simulink model "am_2"  (Simulink 4.00)
settings: Solver=ode45  StartTime=0  StopTime=5  RelTol=1e-3
undefined symbols (not defined in the file or in its folder): B, fmax, fn, Fs, get, k
libraries: dspindex x4, dsparch3 x3, dspsnks3 x3, dspmtrx3 x3, dspsigattribs x2, dspspect3 x2, simulink3 x2, dspbuff3 x2, dspmathops x2, commsource2 x1
Description:
  | Model lacza cyfrowego z modulacja ASK/FSK/PSK
settings Model: Creator=Tomas  LimitDataPoints=off  MaxDataPoints=10000  RTWOptions="-aEnforceIntegerDowncast=1 -aExtMode=0 -aFoldNonRolledExpr=1 -aForceParamTrailComments=0 -aGenerateComments=1 -aIgnoreCustomStorageClasses=1 -aIncHierarchyInIds=0 -aInlineInvariantSignals=0 -aLocalBlockOutputs=1 -aLogVarNameModifier=\"rt_\" -aRTWVerbose=1 -aRollThreshold=5 -aShowEliminatedStatements=1"  RTWInlineParameters=on  BlockReductionOpt=off

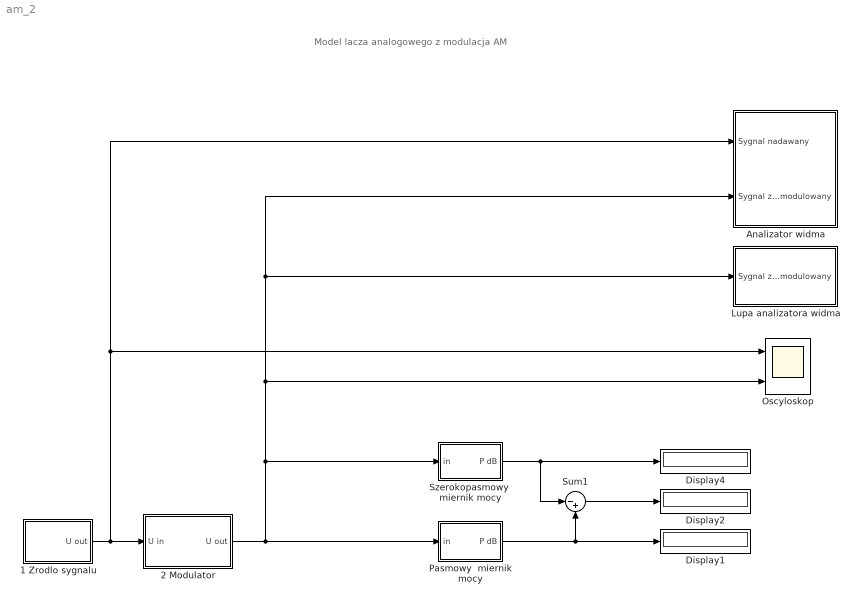
== system am_2 ==
  note: Model lacza analogowego z modulacja AM
  1 Zrodlo sygnalu : Subsystem  mask(Źródło sygnału){on=on, sq=off, bity=100}
      mask prompts: on "Włączenie źródła sygnału"; sq "Przebieg losowy"; bity "częstotliwość/pasmo"
      mask help:
      | Generuje sygnał testowy.
      | Moc wyjściowa 0 dB.
      mask init:
      | if (sq == 0) sq = 1;
      | else sq = 0;
      | end;
      | if (on == 0)
      | set_param(gcb,'MaskEnables',{,'on','off','off'}); fgen=100; G=1;
      | else
      |   set_param(gcb,'MaskEnables',{,'on','on','on'});
      |   if (bity == 1) fgen = 100; G=1/0.1791;
      |   elseif (bity == 2) fgen = 200; G=1/0.2467;
      |   else fgen = 300; G=1/0.3022;
      |   end;
      | end;
      settings: RTWFcnNameOpts=Auto  RTWFileNameOpts=Auto
      mask Help: No help
      mask StyleString: checkbox,checkbox,popup(100|200|300)
      mask Display: disp('Sygnal\nnadawany')
  2 Modulator : Subsystem  mask(Modulator AM){on=on, p=0.7}
      mask prompts: on "Włączenie modulatora"; p "Głębokość modulacji (0..1):"
      mask help:
      | Dokonuje operacji modulacji AM sygnałem podanym na wejście.
      | Częstotliość nośnej: 1000 Hz.
      mask init:
      | fnos=1000;
      | if (on==0) k=1; set_param(gcb,'MaskEnables',{,'on','off'});
      | else set_param(gcb,'MaskEnables',{,'on','on'});
      |   if (p == 1) k = 0.1;
      |   elseif (p == 2) k = 0.2;
      |   elseif (p == 3) k = 0.3;
      |   elseif (p == 4) k = 0.4;
      |   elseif (p == 5) k = 0.5;
      |   elseif (p == 6) k = 0.6;
      |   elseif (p == 7) k = 0.7;
      |   elseif (p == 8) k = 0.8;
      |   elseif (p == 9) k = 0.9;
      |   elseif (p == 10) k = 1.0;
      |   else k = 1.5;
      |   end;
      | end;
      | on=on+1;
      settings: RTWFcnNameOpts=Auto  RTWFileNameOpts=Auto
      mask Help: No help
      mask StyleString: checkbox,popup(0.1|0.2|0.3|0.4|0.5|0.6|0.7|0.8|0.9|1.0|1.5)
      mask Display: disp('Modulator\nAM')
  "Analizator widma " : Subsystem
      settings: RTWFcnNameOpts=Auto  RTWFileNameOpts=Auto
  Display1 : Display
      settings: Format=short
  Display2 : Display
      settings: Format=short
  Display4 : Display
      settings: Format=short
  Lupa analizatora widma : Subsystem  mask(Analizator){f=....fo+1000Hz}
      mask prompts: f "zakres częstotliwości:   fo.."
      mask help: Analizator widma o regulowanym zakresie względem fo=1000Hz
      mask init:
      | if (f==1) fmax=64; elseif (f==2) fmax=128; elseif (f==3) fmax=256; elseif (f==4) fmax=512; else fmax=1024; end;
      settings: RTWFcnNameOpts=Auto  RTWFileNameOpts=Auto
      mask StyleString: popup(....fo+50Hz|....fo+100Hz|....fo+250Hz|....fo+500Hz|....fo+1000Hz)
      mask Display: disp('Lupa')
  Oscyloskop : Scope  NumInputPorts=2
      settings: TimeRange=1  YMin=0~-7.5  YMax=1~7.5  SaveToWorkspace=off  DataFormat=Array  MaxDataPoints=10000
  Pasmowy  miernik mocy : Subsystem  mask(Pasmowy miernik mocy (RMS)){B=200, ca=on, av=on}
      mask prompts: B "pasmo [Hz]"; ca "odfiltruj nośną (1000Hz)"; av "uśrednianie (max. 5 próbek)"
      mask help:
      | Pasmowy miernik mocy (RMS).
      | Częstotliwość środkowa pasma 1000 Hz.
      mask init:
      | fn=1000;
      | BufferSize=4096*8;
      | MaxIndex=BufferSize/2+1;
      | if (B/2<=fn) LowIndex=round(fn-B/2)+1; else LowIndex=1; end;
      | if( B/2+fn<=BufferSize/2) HighIndex=round(fn+B/2)+1; else HighIndex=MaxIndex; end;
      | if (ca==1) ca1_mi_de=round(fn)-3; ca1_pl_de=round(fn)+3;
      | else ca1_mi_de=LowIndex+1; ca1_pl_de=ca1_mi_de+1; end;
      settings: RTWFcnNameOpts=Auto  RTWFileNameOpts=Auto
  Sum1 : Sum  Inputs=|-+  SaturateOnIntegerOverflow=on
  Szerokopasmowy  miernik mocy : Subsystem  mask(Szerokopasmowy miernik mocy (RMS)){ca=on, av=on}
      mask prompts: ca "odfiltruj nośną (1000Hz)"; av "uśrednianie (max 5 próbek)"
      mask help: Szerokopasmowy miernik mocy (RMS).
      mask init:
      | fn=1000;
      | BufferSize=4096*8;
      | MaxIndex=BufferSize/2+1;
      | LowIndex=1;
      | HighIndex=MaxIndex;
      | if (ca==1) ca1_mi_de=round(fn)-3; ca1_pl_de=round(fn)+3;
      | else ca1_mi_de=LowIndex+1; ca1_pl_de=ca1_mi_de+1; end;
      settings: RTWFcnNameOpts=Auto  RTWFileNameOpts=Auto
  wires:
  2 Modulator/1(U out) -> "Analizator widma "/2(Sygnal zmodulowany), Lupa analizatora widma/1(Sygnal zmodulowany), Oscyloskop/2, Szerokopasmowy  miernik mocy/1(in), Pasmowy  miernik mocy/1(in)
  1 Zrodlo sygnalu/1(U out) -> "Analizator widma "/1(Sygnal nadawany), Oscyloskop/1, 2 Modulator/1(U in)
  Sum1/1 -> Display2/1
  Pasmowy  miernik mocy/1(P dB) -> Sum1/2, Display1/1
  Szerokopasmowy  miernik mocy/1(P dB) -> Display4/1, Sum1/1

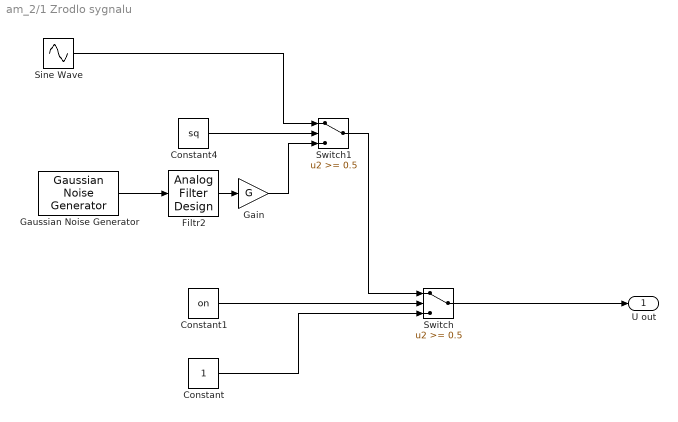
== system am_2/1 Zrodlo sygnalu ==
  Constant : Constant  Value=1
  Constant1 : Constant  Value=on
  Constant4 : Constant  Value=sq
  Filtr2 : dsparch3/Analog Filter Design  method=Chebyshev II  filttype=Lowpass  N=16  Wlo=2*pi*fgen  Whi=2*pi*(fn+B/2)  Rp=2  Rs=60
  Gain : Gain  Gain=G  Multiplication=Element-wise(K.*u)  SaturateOnIntegerOverflow=on
  Gaussian Noise Generator : commsource2/Gaussian Noise Generator  m=0  d=1  s=12345  Ts=1/(6000)  frameBased=off  sampPerFrame=1  orient=off
  Sine Wave : Sin  SineType=Time-based  Amplitude=sqrt(2)  Bias=0  Frequency=2*pi*fgen  Phase=0  Samples=10  SampleTime=0  Offset=0
  Switch : Switch  Threshold=0.5
  Switch1 : Switch  Threshold=0.5
  U out : Outport  Port=1
  wires:
  Switch/1 -> U out/1
  Constant1/1 -> Switch/2
  Switch1/1 -> Switch/1
  Constant4/1 -> Switch1/2
  Sine Wave/1 -> Switch1/1
  Constant/1 -> Switch/3
  Gaussian Noise Generator/1 -> Filtr2/1
  Filtr2/1 -> Gain/1
  Gain/1 -> Switch1/3

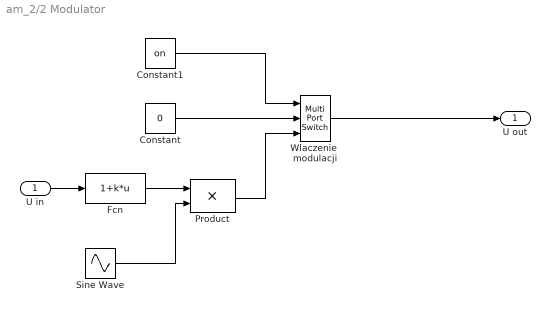
== system am_2/2 Modulator ==
  U in : Inport  Port=1  LatchInput=off
  Constant : Constant  Value=0
  Constant1 : Constant  Value=on
  Fcn : Fcn  Expr=1+k*u
  Product : Product  Inputs=2  Multiplication=Element-wise(.*)  SaturateOnIntegerOverflow=on
  Sine Wave : Sin  SineType=Time-based  Amplitude=1  Bias=0  Frequency=2*pi*1000  Phase=0  Samples=10  SampleTime=0  Offset=0
  Wlaczenie  modulacji : MultiPortSwitch  Inputs=2
  U out : Outport  Port=1
  wires:
  Wlaczenie  modulacji/1 -> U out/1
  Constant1/1 -> Wlaczenie  modulacji/1
  Constant/1 -> Wlaczenie  modulacji/2
  Product/1 -> Wlaczenie  modulacji/3
  U in/1 -> Fcn/1
  Fcn/1 -> Product/1
  Sine Wave/1 -> Product/2

== system am_2/Analizator widma  ==
  Sygnal nadawany : Inport  Port=1  LatchInput=off
  Sygnal zmodulowany : Inport  Port=2  LatchInput=off
  "Sygnal nadawany " : dspsnks3/Spectrum Scope  ScopeProperties=on  Domain=Frequency  HorizSpan=1  UseBuffer=on  BufferSize=4096  Overlap=0  inpFftLenInherit=off  FFTlength=128  numAvg=1  DisplayProperties=off  AxisGrid=on  Memory=on  FrameNumber=off  AxisLegend=off  AxisZoom=off  OpenScopeAtSimStart=on  OpenScopeImmediately=off  FigPos=get(0,'defaultfigureposition')  AxisProperties=off  XUnits=Hertz  XRange=[-Fs/2...Fs/2]  InheritXIncr=on  XIncr=1.0  XLabel=Samples  YUnits=dB  YLabel=Magnitude  LineProperties=off  LineMarkers=None
      settings: YMin=-10  YMax=23.8040697044832
  "Sygnal zmodulowany " : dspsnks3/Spectrum Scope  ScopeProperties=on  Domain=Frequency  HorizSpan=1  UseBuffer=on  BufferSize=4096  Overlap=0  inpFftLenInherit=off  FFTlength=128  numAvg=1  DisplayProperties=off  AxisGrid=on  Memory=on  FrameNumber=off  AxisLegend=off  AxisZoom=off  OpenScopeAtSimStart=on  OpenScopeImmediately=off  FigPos=get(0,'defaultfigureposition')  AxisProperties=off  XUnits=Hertz  XRange=[-Fs/2...Fs/2]  InheritXIncr=on  XIncr=1.0  XLabel=Samples  YUnits=dB  YLabel=Magnitude  LineProperties=off  LineMarkers=None
      settings: YMin=-52.7531800625172  YMax=26.1007017107538
  Unit Delay3 : UnitDelay  X0=0  SampleTime=1/4096
      settings: RTWStateStorageClass=Auto
  Unit Delay4 : UnitDelay  X0=0  SampleTime=1/4096
      settings: RTWStateStorageClass=Auto
  wires:
  Unit Delay4/1 -> "Sygnal nadawany "/1
  Sygnal nadawany/1 -> Unit Delay4/1
  Unit Delay3/1 -> "Sygnal zmodulowany "/1
  Sygnal zmodulowany/1 -> Unit Delay3/1

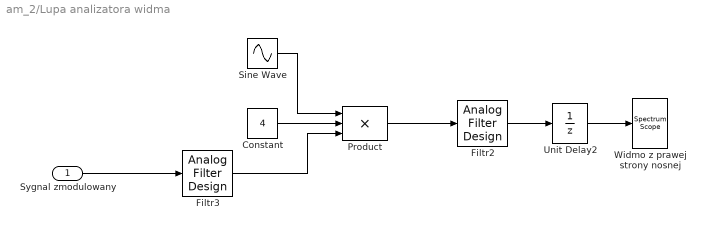
== system am_2/Lupa analizatora widma ==
  Sygnal zmodulowany : Inport  Port=1  LatchInput=off
  Constant : Constant  Value=4
  Filtr2 : dsparch3/Analog Filter Design  method=Elliptic  filttype=Lowpass  N=12  Wlo=2*pi*fmax  Whi=2*pi*(fn+B/2)  Rp=0.2  Rs=80
  Filtr3 : dsparch3/Analog Filter Design  method=Elliptic  filttype=Lowpass  N=26  Wlo=2*pi*1000  Whi=2*pi*(fn+B/2)  Rp=0.2  Rs=80
  Product : Product  Inputs=3  Multiplication=Element-wise(.*)  SaturateOnIntegerOverflow=off
  Sine Wave : Sin  SineType=Time-based  Amplitude=1  Bias=0  Frequency=2*pi*1000  Phase=2*pi-0.03*pi  Samples=10  SampleTime=0  Offset=0
  Unit Delay2 : UnitDelay  X0=0  SampleTime=1/(2*fmax)
      settings: RTWStateStorageClass=Auto
  Widmo z prawej strony nosnej : dspsnks3/Spectrum Scope  ScopeProperties=on  Domain=Frequency  HorizSpan=1  UseBuffer=on  BufferSize=2*fmax  Overlap=0  inpFftLenInherit=off  FFTlength=128  numAvg=1  DisplayProperties=off  AxisGrid=on  Memory=on  FrameNumber=off  AxisLegend=off  AxisZoom=off  OpenScopeAtSimStart=on  OpenScopeImmediately=off  FigPos=get(0,'defaultfigureposition')  AxisProperties=off  XUnits=Hertz  XRange=[0...Fs/2]  InheritXIncr=on  XIncr=1.0  XLabel=Samples  YUnits=dB  YLabel=Magnitude  LineProperties=off  LineMarkers=None
      settings: YMin=-30  YMax=20
  wires:
  Sine Wave/1 -> Product/1
  Product/1 -> Filtr2/1
  Sygnal zmodulowany/1 -> Filtr3/1
  Constant/1 -> Product/2
  Unit Delay2/1 -> Widmo z prawej strony nosnej/1
  Filtr3/1 -> Product/3
  Filtr2/1 -> Unit Delay2/1

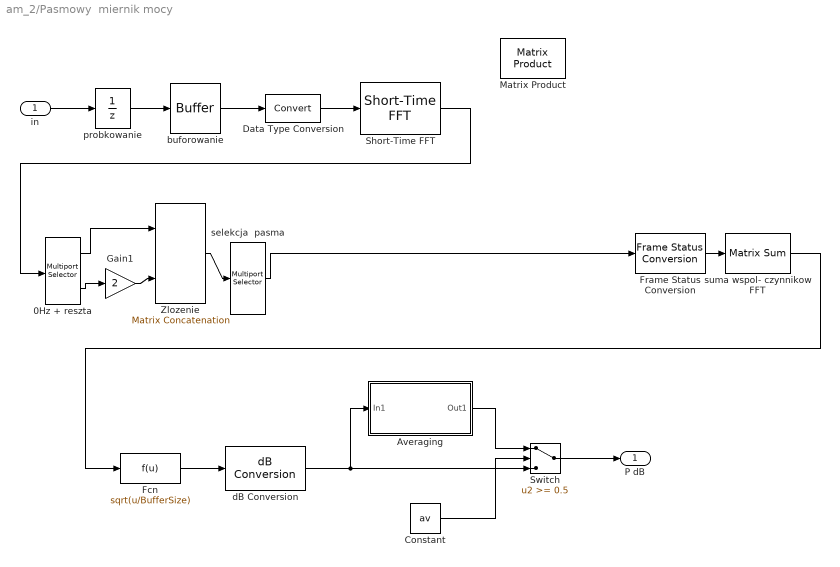
== system am_2/Pasmowy  miernik mocy ==
  in : Inport  Port=1  LatchInput=off
  0Hz + reszta : dspindex/Multiport Selector  rowsOrCols=Rows  idxCellArray={[1],[2:MaxIndex]}  idxErrMode=Generate Error
  Averaging : Subsystem
      settings: RTWFcnNameOpts=Auto  RTWFileNameOpts=Auto
  Constant : Constant  Value=av
  Data Type Conversion : DataTypeConversion  DataType=double  SaturateOnIntegerOverflow=on
  Fcn : Fcn  Expr=sqrt(u/BufferSize)
  Frame Status Conversion : dspsigattribs/Frame Status Conversion  growRefPort=off  outframe=Sample-based
  Gain1 : Gain  Gain=2  Multiplication=Element-wise(K.*u)  SaturateOnIntegerOverflow=on
  Matrix Product : dspmtrx3/Matrix Product  Dim=Columns
  Short-Time FFT : dspspect3/Short-Time FFT  wintype=Hann  Rs=50  beta=5  winsamp=Symmetric  inheritFFT=on  fftsize=FFTlength  navg=1
  Switch : Switch  Threshold=0.5
  Zlozenie : simulink3/Signals & Systems/Matrix Concatenation  numInports=2  catMethod=Vertical
  buforowanie : dspbuff3/Buffer  N=BufferSize  V=0  ic=0
  dB Conversion : dspmathops/dB Conversion  dBtype=dB  intype=Amplitude  R=1  fuzz=on
  probkowanie : UnitDelay  X0=0  SampleTime=1/BufferSize
      settings: RTWStateStorageClass=Auto
  selekcja  pasma : dspindex/Multiport Selector  rowsOrCols=Rows  idxCellArray={[LowIndex:ca1_mi_de ca1_pl_de:HighIndex]}  idxErrMode=Generate Error
  suma wspol- czynnikow FFT : dspmtrx3/Matrix Sum  Dim=Columns
  P dB : Outport  Port=1
  wires:
  Data Type Conversion/1 -> Short-Time FFT/1
  buforowanie/1 -> Data Type Conversion/1
  Frame Status Conversion/1 -> suma wspol- czynnikow FFT/1
  probkowanie/1 -> buforowanie/1
  0Hz + reszta/2 -> Gain1/1
  0Hz + reszta/1 -> Zlozenie/1
  Gain1/1 -> Zlozenie/2
  Zlozenie/1 -> selekcja  pasma/1
  selekcja  pasma/1 -> Frame Status Conversion/1
  Short-Time FFT/1 -> 0Hz + reszta/1
  suma wspol- czynnikow FFT/1 -> Fcn/1
  in/1 -> probkowanie/1
  Fcn/1 -> dB Conversion/1
  Averaging/1(Out1) -> Switch/1
  Switch/1 -> P dB/1
  Constant/1 -> Switch/2
  dB Conversion/1 -> Averaging/1(In1), Switch/3

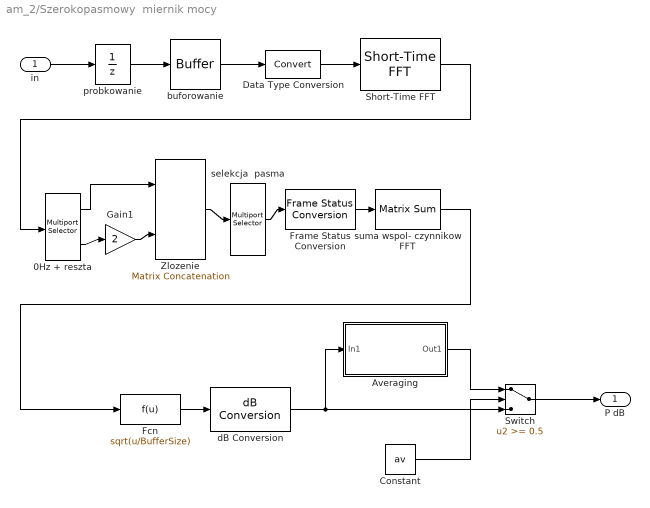
== system am_2/Szerokopasmowy  miernik mocy ==
  in : Inport  Port=1  LatchInput=off
  0Hz + reszta : dspindex/Multiport Selector  rowsOrCols=Rows  idxCellArray={[1],[2:MaxIndex]}  idxErrMode=Generate Error
  Averaging : Subsystem
      settings: RTWFcnNameOpts=Auto  RTWFileNameOpts=Auto
  Constant : Constant  Value=av
  Data Type Conversion : DataTypeConversion  DataType=double  SaturateOnIntegerOverflow=on
  Fcn : Fcn  Expr=sqrt(u/BufferSize)
  Frame Status Conversion : dspsigattribs/Frame Status Conversion  growRefPort=off  outframe=Sample-based
  Gain1 : Gain  Gain=2  Multiplication=Element-wise(K.*u)  SaturateOnIntegerOverflow=on
  Short-Time FFT : dspspect3/Short-Time FFT  wintype=Hann  Rs=50  beta=5  winsamp=Symmetric  inheritFFT=on  fftsize=FFTlength  navg=1
  Switch : Switch  Threshold=0.5
  Zlozenie : simulink3/Signals & Systems/Matrix Concatenation  numInports=2  catMethod=Vertical
  buforowanie : dspbuff3/Buffer  N=BufferSize  V=0  ic=0
  dB Conversion : dspmathops/dB Conversion  dBtype=dB  intype=Amplitude  R=1  fuzz=on
  probkowanie : UnitDelay  X0=0  SampleTime=1/BufferSize
      settings: RTWStateStorageClass=Auto
  selekcja  pasma : dspindex/Multiport Selector  rowsOrCols=Rows  idxCellArray={[LowIndex:ca1_mi_de ca1_pl_de:HighIndex]}  idxErrMode=Generate Error
  suma wspol- czynnikow FFT : dspmtrx3/Matrix Sum  Dim=Columns
  P dB : Outport  Port=1
  wires:
  Data Type Conversion/1 -> Short-Time FFT/1
  buforowanie/1 -> Data Type Conversion/1
  Frame Status Conversion/1 -> suma wspol- czynnikow FFT/1
  probkowanie/1 -> buforowanie/1
  0Hz + reszta/2 -> Gain1/1
  0Hz + reszta/1 -> Zlozenie/1
  Gain1/1 -> Zlozenie/2
  Zlozenie/1 -> selekcja  pasma/1
  selekcja  pasma/1 -> Frame Status Conversion/1
  Short-Time FFT/1 -> 0Hz + reszta/1
  suma wspol- czynnikow FFT/1 -> Fcn/1
  in/1 -> probkowanie/1
  Fcn/1 -> dB Conversion/1
  Averaging/1(Out1) -> Switch/1
  Switch/1 -> P dB/1
  Constant/1 -> Switch/2
  dB Conversion/1 -> Switch/3, Averaging/1(In1)

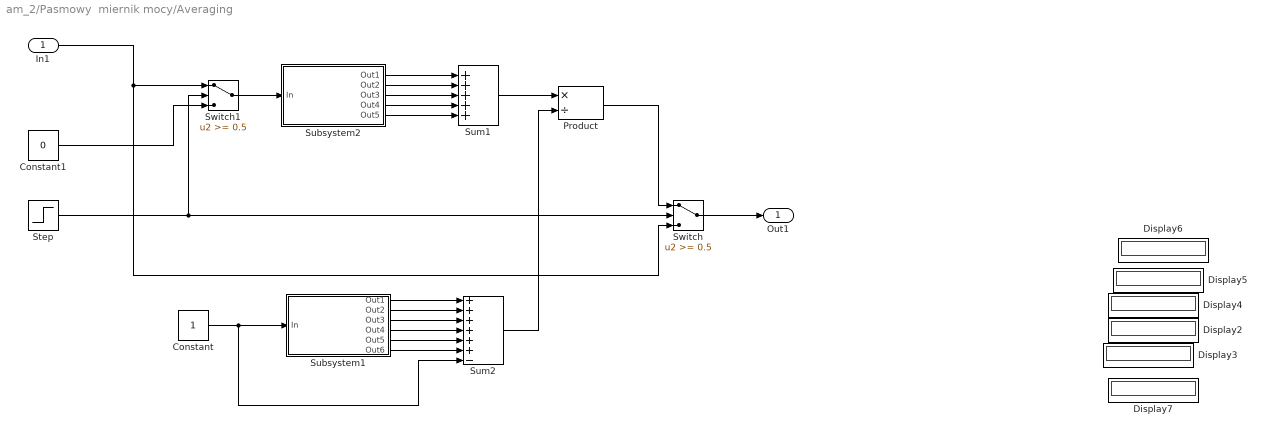
== system am_2/Pasmowy  miernik mocy/Averaging ==
  In1 : Inport  Port=1  LatchInput=off
  Constant : Constant  Value=1
  Constant1 : Constant  Value=0
  Display{2..7} (6 alike) : Display
      settings: Format=short
  Product : Product  Inputs=*/  Multiplication=Element-wise(.*)  SaturateOnIntegerOverflow=on
  Step : Step  Time=1  Before=0  After=1  SampleTime=0
  Subsystem1 : Subsystem  mask(6 Sample Analog Shift Register){tp=1}
      mask prompts: tp "Sample time"
      mask help: 5 Sample Analog Shift Register.
      settings: RTWFcnNameOpts=Auto  RTWFileNameOpts=Auto
      mask Display: disp('6 Sample\nShift\nRegister')
  Subsystem2 : Subsystem  mask(5 Sample Analog Shift Register){tp=1}
      mask prompts: tp "Sample time"
      mask help: 5 Sample Analog Shift Register.
      settings: RTWFcnNameOpts=Auto  RTWFileNameOpts=Auto
      mask Display: disp('5 Sample\nShift\nRegister')
  Sum1 : Sum  Inputs=5  SaturateOnIntegerOverflow=on
  Sum2 : Sum  Inputs=++++++-  SaturateOnIntegerOverflow=on
  Switch : Switch  Threshold=0.5
  Switch1 : Switch  Threshold=0.5
  Out1 : Outport  Port=1
  wires:
  Constant/1 -> Subsystem1/1(In), Sum2/7
  Sum2/1 -> Product/2
  ? -> Display3/1
  ? -> Display2/1
  ? -> Display4/1
  ? -> Display5/1
  ? -> Display6/1
  Subsystem2/1(Out1) -> Sum1/1
  Subsystem2/2(Out2) -> Sum1/2
  Subsystem2/3(Out3) -> Sum1/3
  Subsystem2/4(Out4) -> Sum1/4
  Subsystem2/5(Out5) -> Sum1/5
  Sum1/1 -> Product/1
  Product/1 -> Switch/1
  Step/1 -> Switch/2, Switch1/2
  Switch/1 -> Out1/1
  Subsystem1/1(Out1) -> Sum2/1
  Subsystem1/2(Out2) -> Sum2/2
  Subsystem1/3(Out3) -> Sum2/3
  Subsystem1/4(Out4) -> Sum2/4
  Subsystem1/5(Out5) -> Sum2/5
  Switch1/1 -> Subsystem2/1(In)
  In1/1 -> Switch1/1, Switch/3
  Constant1/1 -> Switch1/3
  Subsystem1/6(Out6) -> Sum2/6

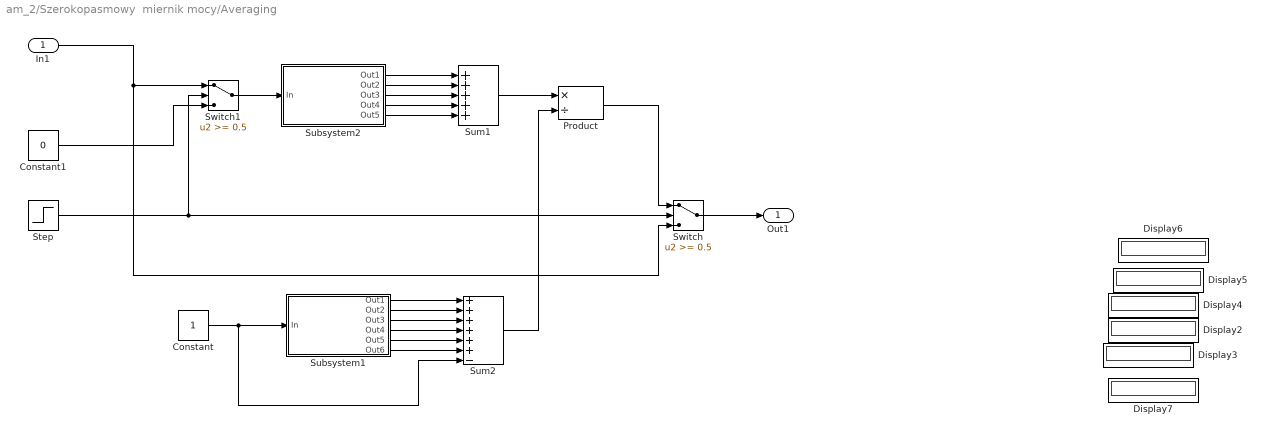
== system am_2/Szerokopasmowy  miernik mocy/Averaging ==
  In1 : Inport  Port=1  LatchInput=off
  Constant : Constant  Value=1
  Constant1 : Constant  Value=0
  Display{2..7} (6 alike) : Display
      settings: Format=short
  Product : Product  Inputs=*/  Multiplication=Element-wise(.*)  SaturateOnIntegerOverflow=on
  Step : Step  Time=1  Before=0  After=1  SampleTime=0
  Subsystem1 : Subsystem  mask(6 Sample Analog Shift Register){tp=1}
      mask prompts: tp "Sample time"
      mask help: 5 Sample Analog Shift Register.
      settings: RTWFcnNameOpts=Auto  RTWFileNameOpts=Auto
      mask Display: disp('6 Sample\nShift\nRegister')
  Subsystem2 : Subsystem  mask(5 Sample Analog Shift Register){tp=1}
      mask prompts: tp "Sample time"
      mask help: 5 Sample Analog Shift Register.
      settings: RTWFcnNameOpts=Auto  RTWFileNameOpts=Auto
      mask Display: disp('5 Sample\nShift\nRegister')
  Sum1 : Sum  Inputs=5  SaturateOnIntegerOverflow=on
  Sum2 : Sum  Inputs=++++++-  SaturateOnIntegerOverflow=on
  Switch : Switch  Threshold=0.5
  Switch1 : Switch  Threshold=0.5
  Out1 : Outport  Port=1
  wires:
  Constant/1 -> Subsystem1/1(In), Sum2/7
  Sum2/1 -> Product/2
  ? -> Display3/1
  ? -> Display2/1
  ? -> Display4/1
  ? -> Display5/1
  ? -> Display6/1
  Subsystem2/1(Out1) -> Sum1/1
  Subsystem2/2(Out2) -> Sum1/2
  Subsystem2/3(Out3) -> Sum1/3
  Subsystem2/4(Out4) -> Sum1/4
  Subsystem2/5(Out5) -> Sum1/5
  Sum1/1 -> Product/1
  Product/1 -> Switch/1
  Step/1 -> Switch/2, Switch1/2
  Switch/1 -> Out1/1
  Subsystem1/1(Out1) -> Sum2/1
  Subsystem1/2(Out2) -> Sum2/2
  Subsystem1/3(Out3) -> Sum2/3
  Subsystem1/4(Out4) -> Sum2/4
  Subsystem1/5(Out5) -> Sum2/5
  Switch1/1 -> Subsystem2/1(In)
  In1/1 -> Switch1/1, Switch/3
  Constant1/1 -> Switch1/3
  Subsystem1/6(Out6) -> Sum2/6

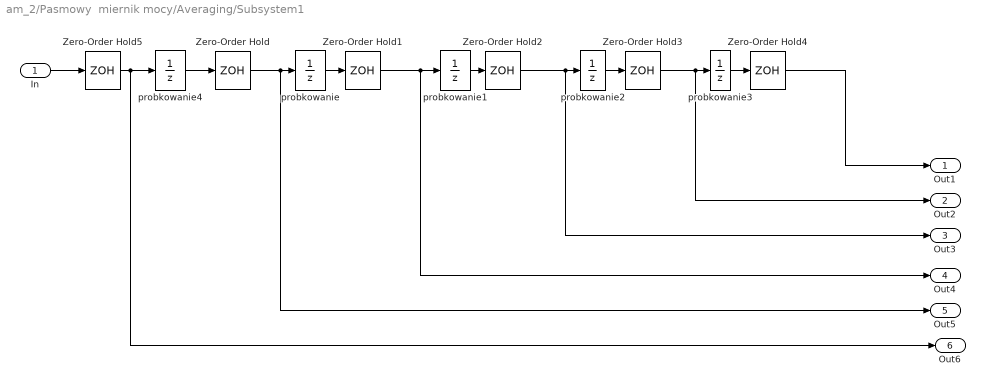
== system am_2/Pasmowy  miernik mocy/Averaging/Subsystem1 ==
  In : Inport  Port=1  LatchInput=off
  Zero-Order Hold{,1..5} (6 alike) : ZeroOrderHold  SampleTime=tp
  probkowanie{,1..4} (5 alike) : UnitDelay  X0=0  SampleTime=0.5*tp
      settings: RTWStateStorageClass=Auto
  Out1 : Outport  Port=1
  Out2 : Outport  Port=2
  Out3 : Outport  Port=3
  Out4 : Outport  Port=4
  Out5 : Outport  Port=5
  Out6 : Outport  Port=6
  wires:
  In/1 -> Zero-Order Hold5/1
  Zero-Order Hold3/1 -> Out2/1, probkowanie3/1
  Zero-Order Hold2/1 -> Out3/1, probkowanie2/1
  Zero-Order Hold1/1 -> Out4/1, probkowanie1/1
  Zero-Order Hold/1 -> Out5/1, probkowanie/1
  Zero-Order Hold4/1 -> Out1/1
  probkowanie/1 -> Zero-Order Hold1/1
  probkowanie1/1 -> Zero-Order Hold2/1
  probkowanie2/1 -> Zero-Order Hold3/1
  probkowanie3/1 -> Zero-Order Hold4/1
  probkowanie4/1 -> Zero-Order Hold/1
  Zero-Order Hold5/1 -> probkowanie4/1, Out6/1

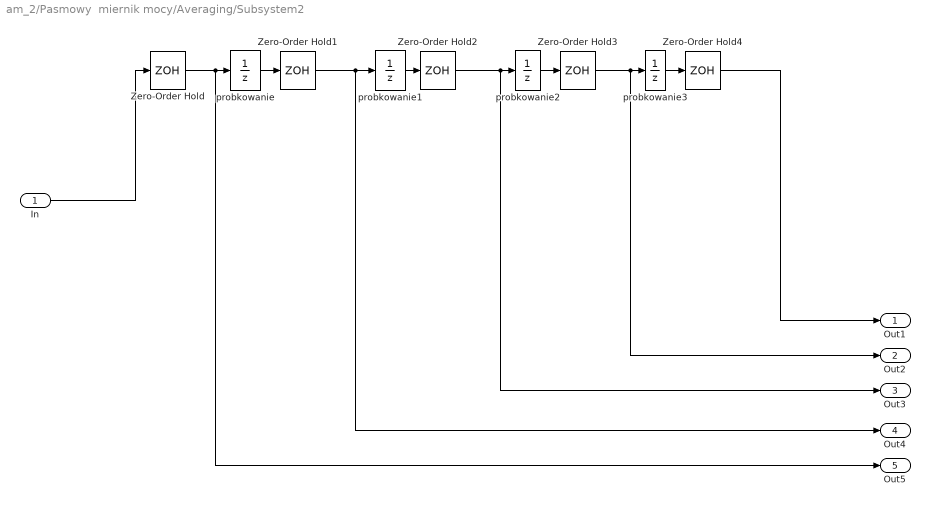
== system am_2/Pasmowy  miernik mocy/Averaging/Subsystem2 ==
  In : Inport  Port=1  LatchInput=off
  Zero-Order Hold{,1..4} (5 alike) : ZeroOrderHold  SampleTime=tp
  probkowanie{,1..3} (4 alike) : UnitDelay  X0=0  SampleTime=0.5*tp
      settings: RTWStateStorageClass=Auto
  Out1 : Outport  Port=1
  Out2 : Outport  Port=2
  Out3 : Outport  Port=3
  Out4 : Outport  Port=4
  Out5 : Outport  Port=5
  wires:
  In/1 -> Zero-Order Hold/1
  Zero-Order Hold3/1 -> Out2/1, probkowanie3/1
  Zero-Order Hold2/1 -> Out3/1, probkowanie2/1
  Zero-Order Hold1/1 -> Out4/1, probkowanie1/1
  Zero-Order Hold/1 -> Out5/1, probkowanie/1
  Zero-Order Hold4/1 -> Out1/1
  probkowanie/1 -> Zero-Order Hold1/1
  probkowanie1/1 -> Zero-Order Hold2/1
  probkowanie2/1 -> Zero-Order Hold3/1
  probkowanie3/1 -> Zero-Order Hold4/1

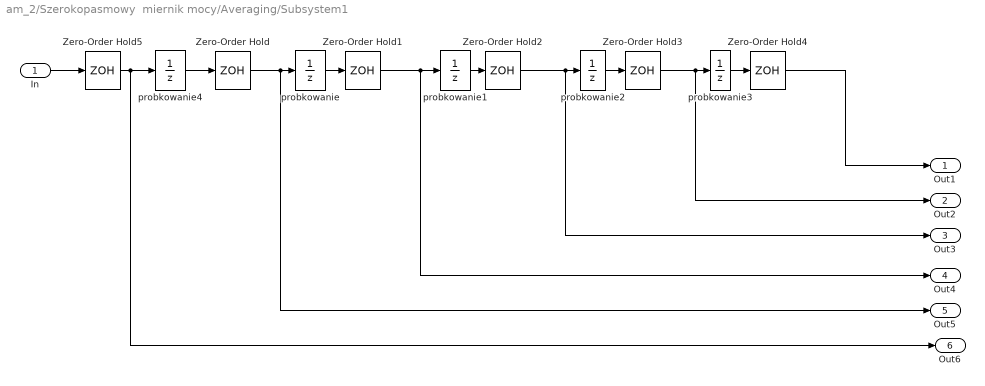
== system am_2/Szerokopasmowy  miernik mocy/Averaging/Subsystem1 ==
  In : Inport  Port=1  LatchInput=off
  Zero-Order Hold{,1..5} (6 alike) : ZeroOrderHold  SampleTime=tp
  probkowanie{,1..4} (5 alike) : UnitDelay  X0=0  SampleTime=0.5*tp
      settings: RTWStateStorageClass=Auto
  Out1 : Outport  Port=1
  Out2 : Outport  Port=2
  Out3 : Outport  Port=3
  Out4 : Outport  Port=4
  Out5 : Outport  Port=5
  Out6 : Outport  Port=6
  wires:
  In/1 -> Zero-Order Hold5/1
  Zero-Order Hold3/1 -> Out2/1, probkowanie3/1
  Zero-Order Hold2/1 -> Out3/1, probkowanie2/1
  Zero-Order Hold1/1 -> Out4/1, probkowanie1/1
  Zero-Order Hold/1 -> Out5/1, probkowanie/1
  Zero-Order Hold4/1 -> Out1/1
  probkowanie/1 -> Zero-Order Hold1/1
  probkowanie1/1 -> Zero-Order Hold2/1
  probkowanie2/1 -> Zero-Order Hold3/1
  probkowanie3/1 -> Zero-Order Hold4/1
  probkowanie4/1 -> Zero-Order Hold/1
  Zero-Order Hold5/1 -> probkowanie4/1, Out6/1

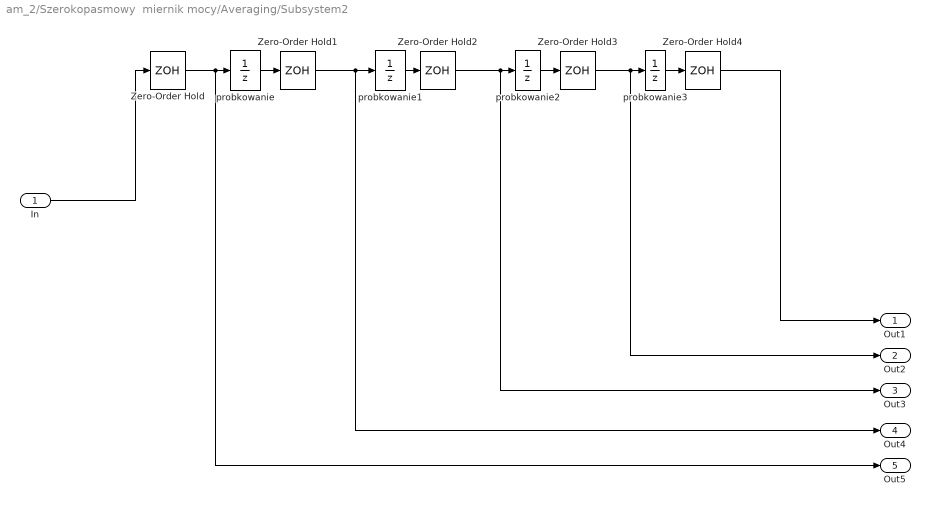
== system am_2/Szerokopasmowy  miernik mocy/Averaging/Subsystem2 ==
  In : Inport  Port=1  LatchInput=off
  Zero-Order Hold{,1..4} (5 alike) : ZeroOrderHold  SampleTime=tp
  probkowanie{,1..3} (4 alike) : UnitDelay  X0=0  SampleTime=0.5*tp
      settings: RTWStateStorageClass=Auto
  Out1 : Outport  Port=1
  Out2 : Outport  Port=2
  Out3 : Outport  Port=3
  Out4 : Outport  Port=4
  Out5 : Outport  Port=5
  wires:
  In/1 -> Zero-Order Hold/1
  Zero-Order Hold3/1 -> Out2/1, probkowanie3/1
  Zero-Order Hold2/1 -> Out3/1, probkowanie2/1
  Zero-Order Hold1/1 -> Out4/1, probkowanie1/1
  Zero-Order Hold/1 -> Out5/1, probkowanie/1
  Zero-Order Hold4/1 -> Out1/1
  probkowanie/1 -> Zero-Order Hold1/1
  probkowanie1/1 -> Zero-Order Hold2/1
  probkowanie2/1 -> Zero-Order Hold3/1
  probkowanie3/1 -> Zero-Order Hold4/1
